simulink model "Ball_and_Beam_grey_box"  (R2018a)
settings: Solver=VariableStepAuto  StartTime=0.0  StopTime=15  RelTol=1e-3
settings Model: Creator=Zeljko  LastModifiedBy=Zeljko

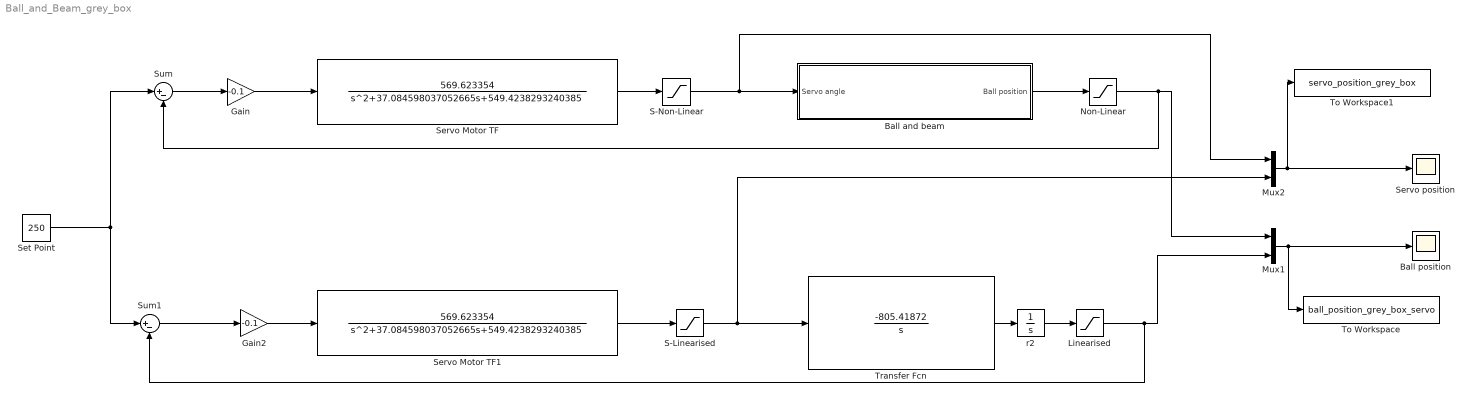
== system Ball_and_Beam_grey_box ==
  Ball and beam : Subsystem
  Ball position : Scope
  Gain : Gain  Gain=-0.1
  Gain2 : Gain  Gain=-0.1
  Linearised : Saturate  UpperLimit=400  LowerLimit=0
  Mux1 : Mux  Inputs=2
  Mux2 : Mux  Inputs=2
  Non-Linear : Saturate  UpperLimit=400  LowerLimit=0
  S-Linearised : Saturate  UpperLimit=45  LowerLimit=-45
  S-Non-Linear : Saturate  UpperLimit=45  LowerLimit=-45
  Servo Motor TF : TransferFcn  Numerator=569.623354  Denominator=[1, 37.084598037052665, 549.4238293240385]
  Servo Motor TF1 : TransferFcn  Numerator=569.623354  Denominator=[1, 37.084598037052665, 549.4238293240385]
  Servo position : Scope
  Set Point : Constant  Value=250
  Sum : Sum  Inputs=|+-
  Sum1 : Sum  Inputs=|+-
  To Workspace : ToWorkspace  VariableName=ball_position_grey_box_servo  SaveFormat=Timeseries  SampleTime=-1
  To Workspace1 : ToWorkspace  VariableName=servo_position_grey_box  SaveFormat=Timeseries  SampleTime=-1
  Transfer Fcn : TransferFcn  Numerator=[-805.41872]  Denominator=[1 0]
  r2 : Integrator  InitialCondition=100
  wires:
  Sum1/1 -> Gain2/1
  Transfer Fcn/1 -> r2/1
  S-Linearised/1 -> Transfer Fcn/1, Mux2/2
  Linearised/1 -> Sum1/2, Mux1/2
  Ball and beam/1(Ball position) -> Non-Linear/1
  Servo Motor TF/1 -> S-Non-Linear/1
  Mux2/1 -> To Workspace1/1, Servo position/1
  Gain/1 -> Servo Motor TF/1
  Non-Linear/1 -> Sum/2, Mux1/1
  Mux1/1 -> To Workspace/1, Ball position/1
  Sum/1 -> Gain/1
  Set Point/1 -> Sum1/1, Sum/1
  Gain2/1 -> Servo Motor TF1/1
  Servo Motor TF1/1 -> S-Linearised/1
  r2/1 -> Linearised/1
  S-Non-Linear/1 -> Mux2/1, Ball and beam/1(Servo angle)

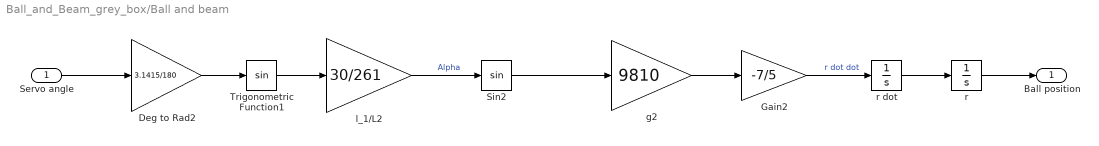
== system Ball_and_Beam_grey_box/Ball and beam ==
  Servo angle : Inport
  Deg to Rad2 : Gain  Gain=3.1415/180
  Gain2 : Gain  Gain=-7/5
  Sin2 : Trigonometry
  Trigonometric Function1 : Trigonometry
  g2 : Gain  Gain=9810
  l_1/L2 : Gain  Gain=30/261
  r : Integrator  InitialCondition=100
  r dot : Integrator
  Ball position : Outport
  wires:
  g2/1 -> Gain2/1
  Sin2/1 -> g2/1
  Deg to Rad2/1 -> Trigonometric Function1/1
  r dot/1 -> r/1
  l_1/L2/1 -> Sin2/1  "Alpha"
  Trigonometric Function1/1 -> l_1/L2/1
  Gain2/1 -> r dot/1  "r dot dot"
  r/1 -> Ball position/1
  Servo angle/1 -> Deg to Rad2/1
